simulink library "variant_3_WEC_Sim_Lib"  (R2014a)
settings: Solver=ode45  StartTime=0.0  StopTime=10.0  RelTol=1e-3
undefined symbols (not defined in the file): body, constraint, pto, simu, waves, X, Y, Z
libraries: nesl_utility x56, sm_lib x43
(part 1 of 2)
settings Model: ForwardingTableString=||__slOldName__||WECSim_Lib/Joints/Translational (heave) PCC||__slNewName__||WECSim_Lib/Joints/Translational (Heave) PCC  Creator=cmichel  LastModifiedBy=cmichel

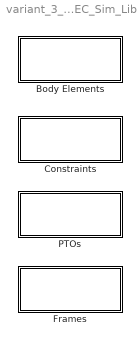
== system variant_3_WEC_Sim_Lib ==
  Body Elements : Subsystem
      mask Display: text(0,0,' ')
  Constraints : Subsystem
      mask Display: text(0,0,' ')
  Frames : Subsystem
      mask Display: text(0,0,' ')
  PTOs : Subsystem
      mask Display: text(0,0,' ')

== system variant_3_WEC_Sim_Lib/Body Elements ==
  Rigid Body : Subsystem  mask(BodyElements){body=body(1)}
      mask prompts: body "Body Name:"
      mask help: This block represents a rigid body. The variable name input below must be 'body(i)' where i=1,2,...
      mask init:
      | if exist('body','var')
      |     h=[gcb '/Structure/Body Properties'];
      |     geomFile=body.geom.file;
      |     set_param(h,'ExtGeomFileName',geomFile);
      |     h=[gcb '/To Workspace'];
      |     responseName=[body.name '_out'];
      |     set_param(h,'VariableName',responseName);
      | end
      | clear bc h geomFile responseName
      settings: AttributesFormatString=%<body>

== system variant_3_WEC_Sim_Lib/Constraints ==
  Fixed : Subsystem  mask(Constraints){constraint=constraint(1)}
      mask prompts: constraint "Constraint Name:"
      mask help:
      | Does not allow any motion. The variable name input below must be 'constraint(i)' where i=1,2,...
      |
      | constraint(i) must be defined in the input file with the following fields:
      |     .name   = a string
      |
      | The name string is used as the variable name for the output power and as such must comply with all of Matlab's variable naming rules.
      mask init:
      | if exist('constraint','var')
      |     h=[gcb '/output'];
      |     responseName=[constraint.name '_out'];
      |     set_param(h,'VariableName',responseName);
      | end
      | 
      | if constraint.loc == [9999 9999 9999]
      |     pto.loc = [0 0 0];
      | end
      settings: AttributesFormatString=%<constraint>
  Floating : Subsystem  mask(Constraints){constraint=constraint(1)}
      mask prompts: constraint "Constraint Name:"
      mask help:
      | Allows body to be free floating (motion in Surge, Heave, and Pitch). The variable name input below must be 'constraint(i)' where i=1,2,...
      |
      | constraint(i) must be defined in the input file with the following fields:
      |     .name   = a string
      |
      | The name string is used as the variable name for the output power and as such must comply with all of Matlab's variable naming rules.
      mask init: same as variant_3_WEC_Sim_Lib/Constraints/Fixed
      settings: AttributesFormatString=%<constraint>
  Heave : Subsystem  mask(Constraints){constraint=constraint(1)}
      mask prompts: constraint "Constraint Name:"
      mask help:
      | Constrains motion to Heave translation only.The variable name input below must be 'constraint(i)' where i=1,2,...
      |
      | constraint(i) must be defined in the input file with the following fields:
      |     .name   = a string
      |
      | The name string is used as the variable name for the output power and as such must comply with all of Matlab's variable naming rules.
      mask init: same as variant_3_WEC_Sim_Lib/Constraints/Fixed
      settings: AttributesFormatString=%<constraint>
  Pitch : Subsystem  mask(Constraints){constraint=constraint(1)}
      mask prompts: constraint "Constraint Name:"
      mask help:
      | Constrains motion to Pitch rotation only. The variable name input below must be 'constraint(i)' where i=1,2,...
      |
      | constraint(i) must be defined in the input file with the following fields:
      |     .name   = a string
      |     .loc    = a 3x1 vector [x y z] in m
      |
      | The name string is used as the variable name for the output power and as such must comply with all of Matlab's variable naming rules.
      mask init:
      | if exist('constraint','var')
      |     h=[gcb '/output'];
      |     responseName=[constraint.name '_out'];
      |     set_param(h,'VariableName',responseName);
      | end
      settings: AttributesFormatString=%<constraint>
  Surge : Subsystem  mask(Constraints){constraint=constraint(1)}
      mask prompts: constraint "Constraint Name:"
      mask help:
      | Constrains motion to Surge translation only.The variable name input below must be 'constraint(i)' where i=1,2,...
      |
      | constraint(i) must be defined in the input file with the following fields:
      |     .name   = a string
      |
      | The name string is used as the variable name for the output power and as such must comply with all of Matlab's variable naming rules.
      mask init: same as variant_3_WEC_Sim_Lib/Constraints/Fixed
      settings: AttributesFormatString=%<constraint>

== system variant_3_WEC_Sim_Lib/Frames ==
  Global Reference Frame : Subsystem  mask(Frames){waves=waves, simu=simu}
      mask prompts: waves "Wave Class Name"; simu "Simulation Class Name"
      mask help:
      | This block contains Global References, including solver configurations, free surface and seabed description, and simulation time.
      | It uses the following fields from the Simulation and Wave classes:
      |
      | Simulation Class:
      |     .endTime
      |     .dt
      |     .domainSize
      |
      | Wave Class:
      |     .waterDepth

== system variant_3_WEC_Sim_Lib/PTOs ==
  External PTO Rotational (Local RY) : Subsystem  mask(External PTO){pto=pto(1)}
      mask prompts: pto "PTO Name:"
      mask help:
      | This PTO constrains the follower (F) to only rotate about the Y-axis of the base (B).
      | The joint is externally actuated (user supplied PTO torque). The joint outputs position and velocity for the user to use in calculating PTO torque.
      mask init:
      | if exist('pto','var')
      |     h=[gcb '/output'];
      |     responseName=[pto.name '_out'];
      |     set_param(h,'VariableName',responseName);
      | end
      settings: AttributesFormatString=%<pto>
  External PTO Translational (Local X) : Subsystem  mask(External PTO){pto=pto(1)}
      mask prompts: pto "PTO Name:"
      mask help:
      | This PTO constrains the follower (F) to only move along the X-direction of the base (B).
      | The joint is externally actuated (user supplied PTO force). The joint outputs position and velocity for the user to use in calculating PTO forces.
      mask init:
      | if exist('pto','var')
      |     h=[gcb '/output'];
      |     responseName=[pto.name '_out'];
      |     set_param(h,'VariableName',responseName);
      | end
      | 
      | if pto.loc == [9999 9999 9999]
      |     pto.loc = [0 0 0];
      | end
      settings: AttributesFormatString=%<pto>
  External PTO Translational (Local Z) : Subsystem  mask(External PTO){pto=pto(1)}
      mask prompts: pto "PTO Name:"
      mask help:
      | This PTO constrains the follower (F) to only move along the Z-direction of the base (B).
      | The joint is externally actuated (user supplied PTO force). The joint outputs position and velocity for the user to use in calculating PTO force.
      mask init:
      | if exist('pto','var')
      |     h=[gcb '/output'];
      |     responseName=[pto.name '_out'];
      |     set_param(h,'VariableName',responseName);
      | end
      | 
      | if pto.loc == [9999 9999 9999]
      |     pto.loc = [0 0 0];
      | end
      settings: AttributesFormatString=%<pto>
  Rotational PTO (Local RY) : Subsystem  mask(PTO){pto=pto(1)}
      mask prompts: pto "PTO Name:"
      mask help:
      | This PTO constrains the follower (F) to only rotate about the Y-axis of the base (B), and applies a PTO stiffness and damping value. The variable name input below must be 'pto(i)' where i=1,2,...
      |
      | pto(i) must be defined in the input file with the following fields:
      |     .name   = a string
      |     .k      = a scalar in N*m/radians
      |     .c      = a scalar in N*m/(radians/s)
      |     .loc    = a 3x1 vector [x y z] in m
      |
      | The name string is used as the variable name for the output power and as such must comply with all of Matlab's variable naming rules.
      mask init:
      | if exist('pto','var')
      |     h=[gcb '/output'];
      |     responseName=[pto.name '_out'];
      |     set_param(h,'VariableName',responseName);
      | end
      settings: AttributesFormatString=%<pto>
  Translational PTO (Local X) : Subsystem  mask(PTO){pto=pto(1)}
      mask prompts: pto "PTO Name:"
      mask help:
      | This PTO constrains the follower (F) to only move along the X-direction of the base (B), and applies a PTO stiffness and damping value. The variable name input below must be 'pto(i)' where i=1,2,...
      |
      | pto(i) must be defined in the input file with the following fields:
      |     .name   = a string
      |     .k      = a scalar in N/m
      |     .c      = a scalar in N/(m/s)
      |
      | The name string is used as the variable name for the output power and as such must comply with all of Matlab's variable naming rules.
      mask init:
      | if exist('pto','var')
      |     h=[gcb '/output'];
      |     responseName=[pto.name '_out'];
      |     set_param(h,'VariableName',responseName);
      | end
      | 
      | if pto.loc == [9999 9999 9999]
      |     pto.loc = [0 0 0];
      | end
      settings: AttributesFormatString=%<pto>
  Translational PTO (Local Z) : Subsystem  mask(PTO){pto=pto(1)}
      mask prompts: pto "PTO Name:"
      mask help:
      | This PTO constrains the follower (F) to only move along the Z-direction of the base (B), and applies a PTO stiffness and damping value. The variable name input below must be 'pto(i)' where i=1,2,...
      |
      | pto(i) must be defined in the input file with the following fields:
      |     .name   = a string
      |     .k      = a scalar in N/m
      |     .c      = a scalar in N/(m/s)
      |
      | The name string is used as the variable name for the output power and as such must comply with all of Matlab's variable naming rules.
      mask init:
      | if exist('pto','var')
      |     h=[gcb '/output'];
      |     responseName=[pto.name '_out'];
      |     set_param(h,'VariableName',responseName);
      | end
      | 
      | if pto.loc == [9999 9999 9999]
      |     pto.loc = [0 0 0];
      | end
      settings: AttributesFormatString=%<pto>

== system variant_3_WEC_Sim_Lib/Body Elements/Rigid Body ==
  Bus Creator : BusCreator  Inputs=5
  Bus Creator1 : BusCreator  Inputs=3
  Bus Selector : BusSelector  OutputSignals=disp,vel,accel
  Bus Selector1 : BusSelector  OutputSignals=F_Excitation,F_Restoring,F_Viscous,F_Mooring,F_Radiation
  Hydrostatic Restoring Force Calculation : Subsystem
  Mooring Force Calculation (Map) : Subsystem
  Structure : Subsystem
  Sum : Sum  Inputs=+----
  To Workspace : ToWorkspace  VariableName=Flap_out  SaveFormat=Structure With Time  SampleTime=-1
  Viscous Damping Force Calculation : Subsystem
  Wave Diffraction and Excitation Force Calculation : Subsystem
  Wave Radiation Forces Calculation : Subsystem
  Conn : PMIOPort  Port=1  Side=Right
  wires:
  Sum/1 -> Bus Creator1/2, Structure/1(F_vector)
  Bus Selector/1 -> Mooring Force Calculation (Map)/1(Displacement), Hydrostatic Restoring Force Calculation/1(Displacement)  "<disp>"
  Bus Selector/2 -> Mooring Force Calculation (Map)/2(Velocity), Viscous Damping Force Calculation/1(Velocity), Wave Radiation Forces Calculation/1(Velocity)  "<vel>"
  Structure/1(Response) -> Bus Selector/1, Bus Creator1/1
  Bus Creator/1 -> Bus Creator1/3, Bus Selector1/1
  Bus Creator1/1 -> To Workspace/1
  Bus Selector/3 -> Wave Radiation Forces Calculation/2(Acceleration)  "<accel>"
  Mooring Force Calculation (Map)/1(F_Mooring) -> Bus Creator/5
  Viscous Damping Force Calculation/1(F_Viscous) -> Bus Creator/4
  Hydrostatic Restoring Force Calculation/1(F_Restoring) -> Bus Creator/3
  Wave Radiation Forces Calculation/1(F_Radiation) -> Bus Creator/2
  Wave Diffraction and Excitation Force Calculation/1(F_Excitation) -> Bus Creator/1
  Bus Selector1/1 -> Sum/1  "<F_Excitation>"
  Bus Selector1/2 -> Sum/2  "<F_Restoring>"
  Bus Selector1/3 -> Sum/3  "<F_Viscous>"
  Bus Selector1/4 -> Sum/4  "<F_Mooring>"
  Bus Selector1/5 -> Sum/5  "<F_Radiation>"
  connections:
  Structure/RConn1 -- Conn/RConn1

== system variant_3_WEC_Sim_Lib/Constraints/Fixed ==
  Mux : Mux  Inputs=2
  PSS : nesl_utility/PS-Simulink Converter  PhysicalDomain=network_engine_domain  SubClassName=ps_output  LeftPortType=input  RightPortType=output  PseudoPeriodic=off  Frequencies=[]  Unit=1  AffineConversion=off
  PSS1 : nesl_utility/PS-Simulink Converter  PhysicalDomain=network_engine_domain  SubClassName=ps_output  LeftPortType=input  RightPortType=output  PseudoPeriodic=off  Frequencies=[]  Unit=1  AffineConversion=off
  Rigid Transform : sm_lib/Frames and Transforms/Rigid Transform  TranslationMethod=Cartesian  TranslationLengthUnit=m  TranslationStandardAxis=+Z  TranslationStandardOffset=0  TranslationCartesianOffset=constraint.loc  TranslationROffset=0  TranslationROffsetUnits=m  TranslationZOffset=0  TranslationZOffsetUnits=m  TranslationThetaOffset=0  TranslationThetaOffsetUnits=deg  RotationMethod=None  RotationAngleUnits=deg  RotationStandardAxis=+X  RotationAngle=90  RotationArbitraryAxis=[0 0 1]  FollAlignAxisA=+X  BaseAlignAxisA=+Y  FollAlignAxisB=+Y  BaseAlignAxisB=+Z  BlockFunction=simmechanics.library.frames_transforms.rigid_transform
  Rigid Transform1 : sm_lib/Frames and Transforms/Rigid Transform  TranslationMethod=Cartesian  TranslationLengthUnit=m  TranslationStandardAxis=+Z  TranslationStandardOffset=0  TranslationCartesianOffset=constraint.loc  TranslationROffset=0  TranslationROffsetUnits=m  TranslationZOffset=0  TranslationZOffsetUnits=m  TranslationThetaOffset=0  TranslationThetaOffsetUnits=deg  RotationMethod=None  RotationAngleUnits=deg  RotationStandardAxis=+X  RotationAngle=90  RotationArbitraryAxis=[0 0 1]  FollAlignAxisA=+X  BaseAlignAxisA=+Y  FollAlignAxisB=+Y  BaseAlignAxisB=+Z  BlockFunction=simmechanics.library.frames_transforms.rigid_transform
  Weld Joint : sm_lib/Joints/Weld Joint  SenseConstraintForce=on  SenseConstraintForceX=off  SenseConstraintForceY=off  SenseConstraintForceZ=off  SenseConstraintTorque=on  SenseConstraintTorqueX=off  SenseConstraintTorqueY=off  SenseConstraintTorqueZ=off  SenseTotalForce=off  SenseTotalForceX=off  SenseTotalForceY=off  SenseTotalForceZ=off  SenseTotalTorque=off  SenseTotalTorqueX=off  SenseTotalTorqueY=off  SenseTotalTorqueZ=off  CompositeWrenchDir=BaseOnFollower  CompositeWrenchFrame=BaseFrame  BlockFunction=simmechanics.library.joints.weld_joint
  output : ToWorkspace  VariableName=Constraint1_out  SaveFormat=Structure With Time  SampleTime=-1
  B : PMIOPort  Port=1  Side=Left
  F : PMIOPort  Port=2  Side=Right
  wires:
  PSS/1 -> Mux/1
  PSS1/1 -> Mux/2
  Mux/1 -> output/1  "Constraint Forces"
  connections:
  PSS1/LConn1 -- Weld Joint/RConn3
  PSS/LConn1 -- Weld Joint/RConn2
  Weld Joint/RConn1 -- Rigid Transform1/RConn1
  Rigid Transform1/LConn1 -- F/RConn1
  Rigid Transform/RConn1 -- Weld Joint/LConn1
  Rigid Transform/LConn1 -- B/RConn1

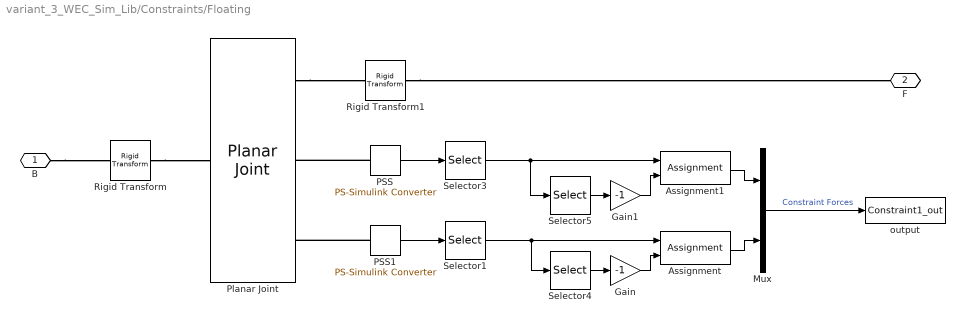
== system variant_3_WEC_Sim_Lib/Constraints/Floating ==
  Assignment : Assignment  DiagnosticForDimensions=Warning  Indices=2
  Assignment1 : Assignment  DiagnosticForDimensions=Warning  Indices=2
  Gain : Gain  Gain=-1
  Gain1 : Gain  Gain=-1
  Mux : Mux  Inputs=2
  PSS : nesl_utility/PS-Simulink Converter  PhysicalDomain=network_engine_domain  SubClassName=ps_output  LeftPortType=input  RightPortType=output  PseudoPeriodic=off  Frequencies=[]  Unit=1  AffineConversion=off
  PSS1 : nesl_utility/PS-Simulink Converter  PhysicalDomain=network_engine_domain  SubClassName=ps_output  LeftPortType=input  RightPortType=output  PseudoPeriodic=off  Frequencies=[]  Unit=1  AffineConversion=off
  Planar Joint : sm_lib/Joints/Planar Joint  SenseConstraintForce=on  SenseConstraintForceX=off  SenseConstraintForceY=off  SenseConstraintForceZ=off  SenseConstraintTorque=on  SenseConstraintTorqueX=off  SenseConstraintTorqueY=off  SenseConstraintTorqueZ=off  SenseTotalForce=off  SenseTotalForceX=off  SenseTotalForceY=off  SenseTotalForceZ=off  SenseTotalTorque=off  SenseTotalTorqueX=off  SenseTotalTorqueY=off  SenseTotalTorqueZ=off  CompositeWrenchDir=BaseOnFollower  CompositeWrenchFrame=BaseFrame  PxEquilibriumPosition=0  PxEquilibriumPositionUnits=m  PxSpringStiffness=0  PxSpringStiffnessUnits=N/m  PxDampingCoefficient=0  PxDampingCoefficientUnits=N/(m/s)  PxTorqueActuationMode=NoTorque  PxMotionActuationMode=ComputedMotion  PxSensePosition=off  PxSenseVelocity=off  PxSenseAcceleration=off  PxSenseTorqueForce=off  PxPositionTargetValue=0  PxPositionTargetValueUnits=m  PxPositionTargetSpecify=off  PxPositionTargetPriority=High  PxVelocityTargetValue=0  PxVelocityTargetValueUnits=m/s  PxVelocityTargetSpecify=off  PxVelocityTargetPriority=High  PyEquilibriumPosition=0  PyEquilibriumPositionUnits=m  PySpringStiffness=0  PySpringStiffnessUnits=N/m  PyDampingCoefficient=0  PyDampingCoefficientUnits=N/(m/s)  PyTorqueActuationMode=NoTorque  PyMotionActuationMode=ComputedMotion  PySensePosition=off  PySenseVelocity=off  PySenseAcceleration=off  PySenseTorqueForce=off  PyPositionTargetValue=0  PyPositionTargetValueUnits=m  PyPositionTargetSpecify=off  PyPositionTargetPriority=High  PyVelocityTargetValue=0  PyVelocityTargetValueUnits=m/s  PyVelocityTargetSpecify=off  PyVelocityTargetPriority=High  RzEquilibriumPosition=0  RzEquilibriumPositionUnits=deg  RzSpringStiffness=0  RzSpringStiffnessUnits=N*m/deg  RzDampingCoefficient=0  RzDampingCoefficientUnits=N*m/(deg/s)  RzTorqueActuationMode=NoTorque  RzMotionActuationMode=ComputedMotion  RzSensePosition=off  RzSenseVelocity=off  RzSenseAcceleration=off  RzSenseTorqueForce=off  RzPositionTargetValue=0  RzPositionTargetValueUnits=deg  RzPositionTargetSpecify=off  RzPositionTargetPriority=High  RzVelocityTargetValue=0  RzVelocityTargetValueUnits=deg/s  RzVelocityTargetSpecify=off  RzVelocityTargetPriority=High  BlockFunction=simmechanics.library.joints.planar_joint
  Rigid Transform : sm_lib/Frames and Transforms/Rigid Transform  TranslationMethod=Cartesian  TranslationLengthUnit=m  TranslationStandardAxis=+Z  TranslationStandardOffset=0  TranslationCartesianOffset=constraint.loc  TranslationROffset=0  TranslationROffsetUnits=m  TranslationZOffset=0  TranslationZOffsetUnits=m  TranslationThetaOffset=0  TranslationThetaOffsetUnits=deg  RotationMethod=StandardAxis  RotationAngleUnits=deg  RotationStandardAxis=+X  RotationAngle=90  RotationArbitraryAxis=[0 0 1]  FollAlignAxisA=+X  BaseAlignAxisA=+Y  FollAlignAxisB=+Y  BaseAlignAxisB=+Z  BlockFunction=simmechanics.library.frames_transforms.rigid_transform
  Rigid Transform1 : sm_lib/Frames and Transforms/Rigid Transform  TranslationMethod=Cartesian  TranslationLengthUnit=m  TranslationStandardAxis=+Z  TranslationStandardOffset=0  TranslationCartesianOffset=constraint.loc  TranslationROffset=0  TranslationROffsetUnits=m  TranslationZOffset=0  TranslationZOffsetUnits=m  TranslationThetaOffset=0  TranslationThetaOffsetUnits=deg  RotationMethod=StandardAxis  RotationAngleUnits=deg  RotationStandardAxis=+X  RotationAngle=90  RotationArbitraryAxis=[0 0 1]  FollAlignAxisA=+X  BaseAlignAxisA=+Y  FollAlignAxisB=+Y  BaseAlignAxisB=+Z  BlockFunction=simmechanics.library.frames_transforms.rigid_transform
  Selector1 : Selector  InputPortWidth=3  Indices=[1 3 2]
  Selector3 : Selector  InputPortWidth=3  Indices=[1 3 2]
  Selector4 : Selector  InputPortWidth=3  Indices=[2]
  Selector5 : Selector  InputPortWidth=3  Indices=[2]
  output : ToWorkspace  VariableName=Constraint1_out  SaveFormat=Structure With Time  SampleTime=-1
  B : PMIOPort  Port=1  Side=Left
  F : PMIOPort  Port=2  Side=Right
  wires:
  Mux/1 -> output/1  "Constraint Forces"
  Selector1/1 -> Assignment/1, Selector4/1
  Selector4/1 -> Gain/1
  Gain/1 -> Assignment/2
  Selector3/1 -> Assignment1/1, Selector5/1
  Selector5/1 -> Gain1/1
  Gain1/1 -> Assignment1/2
  PSS1/1 -> Selector1/1
  PSS/1 -> Selector3/1
  Assignment1/1 -> Mux/1
  Assignment/1 -> Mux/2
  connections:
  Rigid Transform1/LConn1 -- F/RConn1
  Planar Joint/RConn1 -- Rigid Transform1/RConn1
  Rigid Transform/RConn1 -- Planar Joint/LConn1
  B/RConn1 -- Rigid Transform/LConn1
  PSS/LConn1 -- Planar Joint/RConn2
  PSS1/LConn1 -- Planar Joint/RConn3

== system variant_3_WEC_Sim_Lib/Constraints/Heave ==
  Mux : Mux  Inputs=2
  PSS : nesl_utility/PS-Simulink Converter  PhysicalDomain=network_engine_domain  SubClassName=ps_output  LeftPortType=input  RightPortType=output  PseudoPeriodic=off  Frequencies=[]  Unit=1  AffineConversion=off
  PSS1 : nesl_utility/PS-Simulink Converter  PhysicalDomain=network_engine_domain  SubClassName=ps_output  LeftPortType=input  RightPortType=output  PseudoPeriodic=off  Frequencies=[]  Unit=1  AffineConversion=off
  Rigid Transform : sm_lib/Frames and Transforms/Rigid Transform  TranslationMethod=Cartesian  TranslationLengthUnit=m  TranslationStandardAxis=+Z  TranslationStandardOffset=0  TranslationCartesianOffset=constraint.loc  TranslationROffset=0  TranslationROffsetUnits=m  TranslationZOffset=0  TranslationZOffsetUnits=m  TranslationThetaOffset=0  TranslationThetaOffsetUnits=deg  RotationMethod=None  RotationAngleUnits=deg  RotationStandardAxis=+X  RotationAngle=90  RotationArbitraryAxis=[0 0 1]  FollAlignAxisA=+X  BaseAlignAxisA=+Y  FollAlignAxisB=+Y  BaseAlignAxisB=+Z  BlockFunction=simmechanics.library.frames_transforms.rigid_transform
  Rigid Transform1 : sm_lib/Frames and Transforms/Rigid Transform  TranslationMethod=Cartesian  TranslationLengthUnit=m  TranslationStandardAxis=+Z  TranslationStandardOffset=0  TranslationCartesianOffset=constraint.loc  TranslationROffset=0  TranslationROffsetUnits=m  TranslationZOffset=0  TranslationZOffsetUnits=m  TranslationThetaOffset=0  TranslationThetaOffsetUnits=deg  RotationMethod=None  RotationAngleUnits=deg  RotationStandardAxis=+X  RotationAngle=90  RotationArbitraryAxis=[0 0 1]  FollAlignAxisA=+X  BaseAlignAxisA=+Y  FollAlignAxisB=+Y  BaseAlignAxisB=+Z  BlockFunction=simmechanics.library.frames_transforms.rigid_transform
  Translational Constraint (Prismatic Joint) : sm_lib/Joints/Prismatic Joint  SenseConstraintForce=on  SenseConstraintForceX=off  SenseConstraintForceY=off  SenseConstraintForceZ=off  SenseConstraintTorque=on  SenseConstraintTorqueX=off  SenseConstraintTorqueY=off  SenseConstraintTorqueZ=off  SenseTotalForce=off  SenseTotalForceX=off  SenseTotalForceY=off  SenseTotalForceZ=off  SenseTotalTorque=off  SenseTotalTorqueX=off  SenseTotalTorqueY=off  SenseTotalTorqueZ=off  CompositeWrenchDir=BaseOnFollower  CompositeWrenchFrame=BaseFrame  EquilibriumPosition=0  EquilibriumPositionUnits=m  SpringStiffness=0  SpringStiffnessUnits=N/m  DampingCoefficient=0  DampingCoefficientUnits=N/(m/s)  TorqueActuationMode=NoTorque  MotionActuationMode=ComputedMotion  SensePosition=off  SenseVelocity=off  SenseAcceleration=off  SenseTorqueForce=off  PositionTargetValue=0  PositionTargetValueUnits=m  PositionTargetSpecify=off  PositionTargetPriority=High  VelocityTargetValue=0  VelocityTargetValueUnits=m/s  VelocityTargetSpecify=off  VelocityTargetPriority=High  BlockFunction=simmechanics.library.joints.prismatic_joint
  output : ToWorkspace  VariableName=Constraint1_out  SaveFormat=Structure With Time  SampleTime=-1
  F : PMIOPort  Port=1  Side=Right
  B : PMIOPort  Port=2  Side=Left
  wires:
  PSS/1 -> Mux/1
  PSS1/1 -> Mux/2
  Mux/1 -> output/1  "Constraint Forces"
  connections:
  PSS/LConn1 -- Translational Constraint (Prismatic Joint)/RConn2
  PSS1/LConn1 -- Translational Constraint (Prismatic Joint)/RConn3
  Translational Constraint (Prismatic Joint)/RConn1 -- Rigid Transform1/RConn1
  Rigid Transform1/LConn1 -- F/RConn1
  B/RConn1 -- Rigid Transform/LConn1
  Rigid Transform/RConn1 -- Translational Constraint (Prismatic Joint)/LConn1

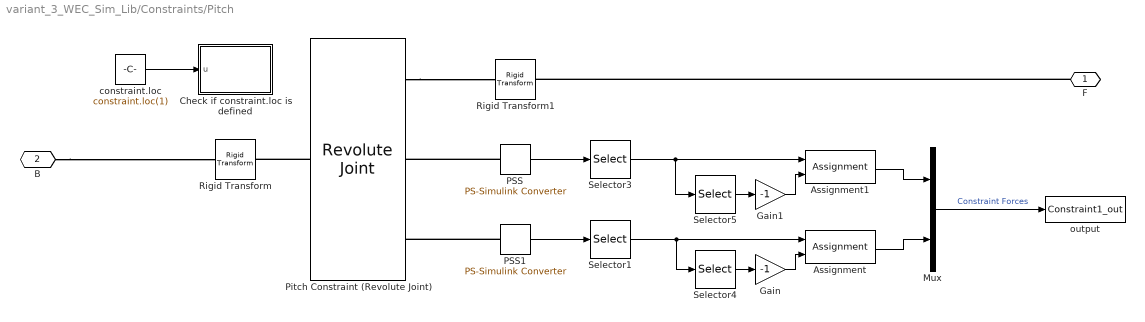
== system variant_3_WEC_Sim_Lib/Constraints/Pitch ==
  Assignment : Assignment  DiagnosticForDimensions=Warning  Indices=2
  Assignment1 : Assignment  DiagnosticForDimensions=Warning  Indices=2
  "Check if constraint.loc is defined " : MATLAB Function  TreatAsAtomicUnit=on
  Gain : Gain  Gain=-1
  Gain1 : Gain  Gain=-1
  Mux : Mux  Inputs=2
  PSS : nesl_utility/PS-Simulink Converter  PhysicalDomain=network_engine_domain  SubClassName=ps_output  LeftPortType=input  RightPortType=output  PseudoPeriodic=off  Frequencies=[]  Unit=1  AffineConversion=off
  PSS1 : nesl_utility/PS-Simulink Converter  PhysicalDomain=network_engine_domain  SubClassName=ps_output  LeftPortType=input  RightPortType=output  PseudoPeriodic=off  Frequencies=[]  Unit=1  AffineConversion=off
  Pitch Constraint (Revolute Joint) : sm_lib/Joints/Revolute Joint  SenseConstraintForce=on  SenseConstraintForceX=off  SenseConstraintForceY=off  SenseConstraintForceZ=off  SenseConstraintTorque=on  SenseConstraintTorqueX=off  SenseConstraintTorqueY=off  SenseConstraintTorqueZ=off  SenseTotalForce=off  SenseTotalForceX=off  SenseTotalForceY=off  SenseTotalForceZ=off  SenseTotalTorque=off  SenseTotalTorqueX=off  SenseTotalTorqueY=off  SenseTotalTorqueZ=off  CompositeWrenchDir=BaseOnFollower  CompositeWrenchFrame=BaseFrame  EquilibriumPosition=0  EquilibriumPositionUnits=deg  SpringStiffness=0  SpringStiffnessUnits=N*m/deg  DampingCoefficient=0  DampingCoefficientUnits=N*m/(rad/s)  TorqueActuationMode=NoTorque  MotionActuationMode=ComputedMotion  SensePosition=off  SenseVelocity=off  SenseAcceleration=off  SenseTorqueForce=off  PositionTargetValue=0  PositionTargetValueUnits=deg  PositionTargetSpecify=off  PositionTargetPriority=High  VelocityTargetValue=0  VelocityTargetValueUnits=deg/s  VelocityTargetSpecify=off  VelocityTargetPriority=High  BlockFunction=simmechanics.library.joints.revolute_joint
  Rigid Transform : sm_lib/Frames and Transforms/Rigid Transform  TranslationMethod=Cartesian  TranslationLengthUnit=m  TranslationStandardAxis=+Z  TranslationStandardOffset=0  TranslationCartesianOffset=constraint.loc  TranslationROffset=0  TranslationROffsetUnits=m  TranslationZOffset=0  TranslationZOffsetUnits=m  TranslationThetaOffset=0  TranslationThetaOffsetUnits=deg  RotationMethod=StandardAxis  RotationAngleUnits=deg  RotationStandardAxis=+X  RotationAngle=90  RotationArbitraryAxis=[0 0 1]  FollAlignAxisA=+X  BaseAlignAxisA=+Y  FollAlignAxisB=+Y  BaseAlignAxisB=+Z  BlockFunction=simmechanics.library.frames_transforms.rigid_transform
  Rigid Transform1 : sm_lib/Frames and Transforms/Rigid Transform  TranslationMethod=Cartesian  TranslationLengthUnit=m  TranslationStandardAxis=+Z  TranslationStandardOffset=0  TranslationCartesianOffset=constraint.loc  TranslationROffset=0  TranslationROffsetUnits=m  TranslationZOffset=0  TranslationZOffsetUnits=m  TranslationThetaOffset=0  TranslationThetaOffsetUnits=deg  RotationMethod=StandardAxis  RotationAngleUnits=deg  RotationStandardAxis=+X  RotationAngle=90  RotationArbitraryAxis=[0 0 1]  FollAlignAxisA=+X  BaseAlignAxisA=+Y  FollAlignAxisB=+Y  BaseAlignAxisB=+Z  BlockFunction=simmechanics.library.frames_transforms.rigid_transform
  Selector1 : Selector  InputPortWidth=3  Indices=[1 3 2]
  Selector3 : Selector  InputPortWidth=3  Indices=[1 3 2]
  Selector4 : Selector  InputPortWidth=3  Indices=[2]
  Selector5 : Selector  InputPortWidth=3  Indices=[2]
  constraint.loc : Constant  Value=constraint.loc(1)  VectorParams1D=off
  output : ToWorkspace  VariableName=Constraint1_out  SaveFormat=Structure With Time  SampleTime=-1
  F : PMIOPort  Port=1  Side=Right
  B : PMIOPort  Port=2  Side=Left
  wires:
  Mux/1 -> output/1  "Constraint Forces"
  constraint.loc/1 -> "Check if constraint.loc is defined "/1(u)
  PSS/1 -> Selector3/1
  PSS1/1 -> Selector1/1
  Selector1/1 -> Assignment/1, Selector4/1
  Selector4/1 -> Gain/1
  Gain/1 -> Assignment/2
  Assignment/1 -> Mux/2
  Selector3/1 -> Assignment1/1, Selector5/1
  Selector5/1 -> Gain1/1
  Gain1/1 -> Assignment1/2
  Assignment1/1 -> Mux/1
  connections:
  Pitch Constraint (Revolute Joint)/LConn1 -- Rigid Transform/RConn1
  Pitch Constraint (Revolute Joint)/RConn1 -- Rigid Transform1/RConn1
  B/RConn1 -- Rigid Transform/LConn1
  F/RConn1 -- Rigid Transform1/LConn1
  PSS/LConn1 -- Pitch Constraint (Revolute Joint)/RConn2
  PSS1/LConn1 -- Pitch Constraint (Revolute Joint)/RConn3

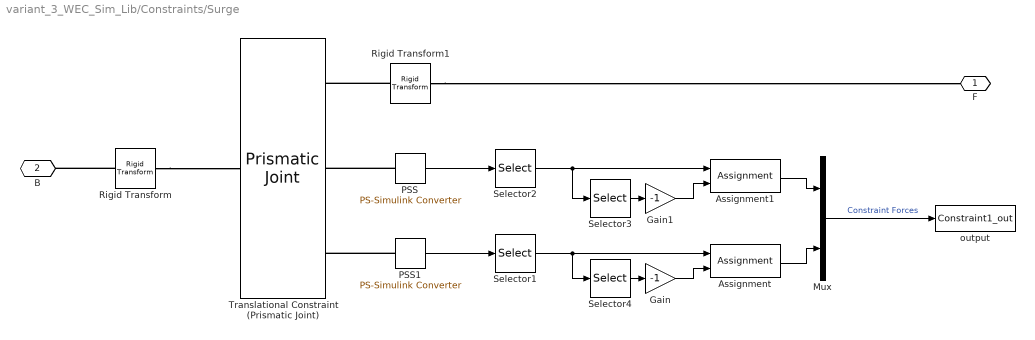
== system variant_3_WEC_Sim_Lib/Constraints/Surge ==
  Assignment : Assignment  DiagnosticForDimensions=Warning  Indices=3
  Assignment1 : Assignment  DiagnosticForDimensions=Warning  Indices=3
  Gain : Gain  Gain=-1
  Gain1 : Gain  Gain=-1
  Mux : Mux  Inputs=2
  PSS : nesl_utility/PS-Simulink Converter  PhysicalDomain=network_engine_domain  SubClassName=ps_output  LeftPortType=input  RightPortType=output  PseudoPeriodic=off  Frequencies=[]  Unit=1  AffineConversion=off
  PSS1 : nesl_utility/PS-Simulink Converter  PhysicalDomain=network_engine_domain  SubClassName=ps_output  LeftPortType=input  RightPortType=output  PseudoPeriodic=off  Frequencies=[]  Unit=1  AffineConversion=off
  Rigid Transform : sm_lib/Frames and Transforms/Rigid Transform  TranslationMethod=Cartesian  TranslationLengthUnit=m  TranslationStandardAxis=+Z  TranslationStandardOffset=0  TranslationCartesianOffset=constraint.loc  TranslationROffset=0  TranslationROffsetUnits=m  TranslationZOffset=0  TranslationZOffsetUnits=m  TranslationThetaOffset=0  TranslationThetaOffsetUnits=deg  RotationMethod=StandardAxis  RotationAngleUnits=deg  RotationStandardAxis=+Y  RotationAngle=90  RotationArbitraryAxis=[0 0 1]  FollAlignAxisA=+X  BaseAlignAxisA=+Y  FollAlignAxisB=+Y  BaseAlignAxisB=+Z  BlockFunction=simmechanics.library.frames_transforms.rigid_transform
  Rigid Transform1 : sm_lib/Frames and Transforms/Rigid Transform  TranslationMethod=Cartesian  TranslationLengthUnit=m  TranslationStandardAxis=+Z  TranslationStandardOffset=0  TranslationCartesianOffset=constraint.loc  TranslationROffset=0  TranslationROffsetUnits=m  TranslationZOffset=0  TranslationZOffsetUnits=m  TranslationThetaOffset=0  TranslationThetaOffsetUnits=deg  RotationMethod=StandardAxis  RotationAngleUnits=deg  RotationStandardAxis=+Y  RotationAngle=90  RotationArbitraryAxis=[0 0 1]  FollAlignAxisA=+X  BaseAlignAxisA=+Y  FollAlignAxisB=+Y  BaseAlignAxisB=+Z  BlockFunction=simmechanics.library.frames_transforms.rigid_transform
  Selector1 : Selector  InputPortWidth=3  Indices=[3 2 1]
  Selector2 : Selector  InputPortWidth=3  Indices=[3 2 1]
  Selector3 : Selector  InputPortWidth=3  Indices=[3]
  Selector4 : Selector  InputPortWidth=3  Indices=[3]
  Translational Constraint (Prismatic Joint) : sm_lib/Joints/Prismatic Joint  SenseConstraintForce=on  SenseConstraintForceX=off  SenseConstraintForceY=off  SenseConstraintForceZ=off  SenseConstraintTorque=on  SenseConstraintTorqueX=off  SenseConstraintTorqueY=off  SenseConstraintTorqueZ=off  SenseTotalForce=off  SenseTotalForceX=off  SenseTotalForceY=off  SenseTotalForceZ=off  SenseTotalTorque=off  SenseTotalTorqueX=off  SenseTotalTorqueY=off  SenseTotalTorqueZ=off  CompositeWrenchDir=BaseOnFollower  CompositeWrenchFrame=BaseFrame  EquilibriumPosition=0  EquilibriumPositionUnits=m  SpringStiffness=0  SpringStiffnessUnits=N/m  DampingCoefficient=0  DampingCoefficientUnits=N/(m/s)  TorqueActuationMode=NoTorque  MotionActuationMode=ComputedMotion  SensePosition=off  SenseVelocity=off  SenseAcceleration=off  SenseTorqueForce=off  PositionTargetValue=0  PositionTargetValueUnits=m  PositionTargetSpecify=off  PositionTargetPriority=High  VelocityTargetValue=0  VelocityTargetValueUnits=m/s  VelocityTargetSpecify=off  VelocityTargetPriority=High  BlockFunction=simmechanics.library.joints.prismatic_joint
  output : ToWorkspace  VariableName=Constraint1_out  SaveFormat=Structure With Time  SampleTime=-1
  F : PMIOPort  Port=1  Side=Right
  B : PMIOPort  Port=2  Side=Left
  wires:
  Mux/1 -> output/1  "Constraint Forces"
  Selector1/1 -> Assignment/1, Selector4/1
  Selector4/1 -> Gain/1
  Gain/1 -> Assignment/2
  PSS1/1 -> Selector1/1
  Selector2/1 -> Assignment1/1, Selector3/1
  Selector3/1 -> Gain1/1
  Gain1/1 -> Assignment1/2
  PSS/1 -> Selector2/1
  Assignment1/1 -> Mux/1
  Assignment/1 -> Mux/2
  connections:
  Rigid Transform1/LConn1 -- F/RConn1
  Rigid Transform1/RConn1 -- Translational Constraint (Prismatic Joint)/RConn1
  Rigid Transform/RConn1 -- Translational Constraint (Prismatic Joint)/LConn1
  Rigid Transform/LConn1 -- B/RConn1
  PSS/LConn1 -- Translational Constraint (Prismatic Joint)/RConn2
  PSS1/LConn1 -- Translational Constraint (Prismatic Joint)/RConn3

== system variant_3_WEC_Sim_Lib/Frames/Global Reference Frame ==
  note: NOTE:Must be a fixed time step solver
      | changed to ode4 (fixed step)
  Clock : Clock
  Mean Free Surface : sm_lib/Body Elements/Solid  InertiaType=Custom  Mass=10^20  MassUnits=kg  CenterOfMass=[0 0 0]  CenterOfMassUnits=m  MomentsOfInertia=[10^20 10^20 10^20]  MomentsOfInertiaUnits=kg*m^2  ProductsOfInertia=[0 0 0]  ProductsOfInertiaUnits=kg*m^2  DensityBased=on  Density=1000  DensityUnits=kg/(m^3)  GraphicType=FromGeometry  MarkerShape=Sphere  MarkerSize=10  MarkerSizeUnits=m  GraphicVisPropType=SimpleVisualProperties  GraphicDiffuseColor=[0.0 0.6 0.8]  GraphicSpecularColor=[0.5 0.5 0.5 1.0]  GraphicAmbientColor=[0.15 0.15 0.15 1.0]  GraphicEmissiveColor=[0.0 0.0 0.0 1.0]  GraphicShininess=75  GraphicOpacity=0.3  GeometryShape=GeneralExtrusion  RectangleSize=[1 1]  RectangleSizeUnits=m  BrickDimensions=[1 1 1]  BrickDimensionUnits=m  CylinderRadius=1  CylinderRadiusUnits=m  CylinderLength=1  CylinderLengthUnits=m  SphereRadius=1  SphereRadiusUnits=m  EllipsoidRadii=[1 1 1]  EllipsoidRadiiUnits=m  ExtrusionCrossSection=[simu.domainSize simu.domainSize; -simu.domainSize simu.domainSize; -simu.domainSize -simu.domainSize; simu.domainSize -simu.domainSize]  ExtrusionCrossSectionUnits=m  ExtrusionLength=simu.domainSize/200  ExtrusionLengthUnits=m  PolygonNumSides=3  PolygonOuterRadius=1  PolygonOuterRadiusUnits=m  ExtGeomFileType=STL  ExtGeomFileUnits=m  RevolutionCrossSection=[1 1; 1 -1; 2 -1; 2 1]  RevolutionCrossSectionUnits=m  RevolutionExtent=Full  RevolutionAngle=180  RevolutionAngleUnits=deg  BlockFunction=simmechanics.library.body_elements.solid
  Mechanism Configuration1 : sm_lib/Utilities/Mechanism Configuration  UniformGravity=Constant  GravityVector=[0 0 0]  GravityUnits=m/s^2  LinearizationDelta=0.001  BlockFunction=simmechanics.library.utilities.mechanism_configuration
  Rigid Transform : sm_lib/Frames and Transforms/Rigid Transform  TranslationMethod=Cartesian  TranslationLengthUnit=m  TranslationStandardAxis=+Z  TranslationStandardOffset=0  TranslationCartesianOffset=[0 0 -waves.waterDepth]  TranslationROffset=0  TranslationROffsetUnits=m  TranslationZOffset=0  TranslationZOffsetUnits=m  TranslationThetaOffset=0  TranslationThetaOffsetUnits=deg  RotationMethod=None  RotationAngleUnits=deg  RotationStandardAxis=+Z  RotationAngle=0  RotationArbitraryAxis=[0 0 1]  FollAlignAxisA=+X  BaseAlignAxisA=+Y  FollAlignAxisB=+Y  BaseAlignAxisB=+Z  BlockFunction=simmechanics.library.frames_transforms.rigid_transform
  Seabed : sm_lib/Body Elements/Solid  InertiaType=Custom  Mass=10^20  MassUnits=kg  CenterOfMass=[0 0 0]  CenterOfMassUnits=m  MomentsOfInertia=[10^20 10^20 10^20]  MomentsOfInertiaUnits=kg*m^2  ProductsOfInertia=[0 0 0]  ProductsOfInertiaUnits=kg*m^2  DensityBased=on  Density=1000  DensityUnits=kg/(m^3)  GraphicType=FromGeometry  MarkerShape=Sphere  MarkerSize=10  MarkerSizeUnits=m  GraphicVisPropType=SimpleVisualProperties  GraphicDiffuseColor=[0.4 0.4 0.0]  GraphicSpecularColor=[0.5 0.5 0.5 1.0]  GraphicAmbientColor=[0.15 0.15 0.15 1.0]  GraphicEmissiveColor=[0.0 0.0 0.0 1.0]  GraphicShininess=75  GraphicOpacity=1  GeometryShape=GeneralExtrusion  RectangleSize=[1 1]  RectangleSizeUnits=m  BrickDimensions=[1 1 1]  BrickDimensionUnits=m  CylinderRadius=1  CylinderRadiusUnits=m  CylinderLength=1  CylinderLengthUnits=m  SphereRadius=1  SphereRadiusUnits=m  EllipsoidRadii=[1 1 1]  EllipsoidRadiiUnits=m  ExtrusionCrossSection=[simu.domainSize simu.domainSize; -simu.domainSize simu.domainSize; -simu.domainSize -simu.domainSize; simu.domainSize -simu.domainSize]  ExtrusionCrossSectionUnits=m  ExtrusionLength=simu.domainSize/100  ExtrusionLengthUnits=m  PolygonNumSides=3  PolygonOuterRadius=1  PolygonOuterRadiusUnits=m  ExtGeomFileType=STL  ExtGeomFileUnits=m  RevolutionCrossSection=[1 1; 1 -1; 2 -1; 2 1]  RevolutionCrossSectionUnits=m  RevolutionExtent=Full  RevolutionAngle=180  RevolutionAngleUnits=deg  BlockFunction=simmechanics.library.body_elements.solid
  Solver Configuration : nesl_utility/Solver Configuration  PhysicalDomain=network_engine_domain  SubClassName=solver  LeftPortType=input  RightPortType=generic  Accelerate=off  Tones=[]  Harmonics=[]  SimulateNoise=off  Profile=off  UseLocalSampling=off  EnableSwitchedLinearOptims=on  FrequencyDomain=off  UseCCode=off  RelTol=0.001  AbsTol=1e-06  MinStep=1e-09  ToWorkspace=off  DoDC=on  ResidualTolerance=1e-9  UseLocalSolver=off  LocalSolverChoice=NE_BACKWARD_EULER_ADVANCER  LocalSolverSampleTime=.001  DoFixedCost=off  MaxNonlinIter=3  MaxModeIter=2  LinearAlgebra=Sparse  DelaysMemoryBudget=1024  AutomaticFiltering=on  FilteringTimeConstant=0.001
  World Frame2 : sm_lib/Frames and Transforms/World Frame  BlockFunction=simmechanics.library.frames_transforms.world_frame
  Conn : PMIOPort  Port=1  Side=Right
  tag scope: Clock=global
  wires:
  Clock/1 -> [Clock]
  connections:
  Mechanism Configuration1/RConn1 -- World Frame2/RConn1 -- Solver Configuration/RConn1 -- Mean Free Surface/RConn1 -- Rigid Transform/LConn1 -- Conn/RConn1
  Seabed/RConn1 -- Rigid Transform/RConn1

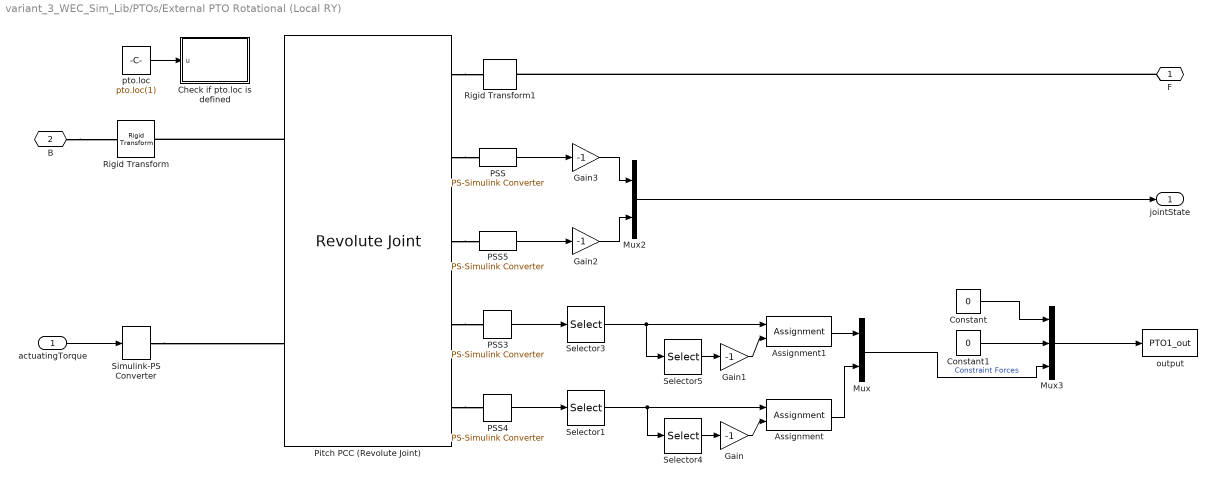
== system variant_3_WEC_Sim_Lib/PTOs/External PTO Rotational (Local RY) ==
  actuatingTorque : Inport
  Assignment : Assignment  DiagnosticForDimensions=Warning  Indices=2
  Assignment1 : Assignment  DiagnosticForDimensions=Warning  Indices=2
  "Check if pto.loc is defined " : MATLAB Function  TreatAsAtomicUnit=on
  Constant : Constant  Value=0
  Constant1 : Constant  Value=0
  Gain{,1..3} (4 alike) : Gain  Gain=-1
  Mux : Mux  Inputs=2
  Mux2 : Mux  Inputs=2
  Mux3 : Mux  Inputs=3
  PSS{,3..5} (4 alike) : nesl_utility/PS-Simulink Converter  PhysicalDomain=network_engine_domain  SubClassName=ps_output  LeftPortType=input  RightPortType=output  PseudoPeriodic=off  Frequencies=[]  Unit=1  AffineConversion=off
  Pitch PCC (Revolute Joint) : sm_lib/Joints/Revolute Joint  SenseConstraintForce=on  SenseConstraintForceX=off  SenseConstraintForceY=off  SenseConstraintForceZ=off  SenseConstraintTorque=on  SenseConstraintTorqueX=off  SenseConstraintTorqueY=off  SenseConstraintTorqueZ=off  SenseTotalForce=off  SenseTotalForceX=off  SenseTotalForceY=off  SenseTotalForceZ=off  SenseTotalTorque=off  SenseTotalTorqueX=off  SenseTotalTorqueY=off  SenseTotalTorqueZ=off  CompositeWrenchDir=BaseOnFollower  CompositeWrenchFrame=BaseFrame  EquilibriumPosition=0  EquilibriumPositionUnits=deg  SpringStiffness=0  SpringStiffnessUnits=N*m/rad  DampingCoefficient=0  DampingCoefficientUnits=N*m/(rad/s)  TorqueActuationMode=InputTorque  MotionActuationMode=ComputedMotion  SensePosition=on  SenseVelocity=on  SenseAcceleration=off  SenseTorqueForce=off  PositionTargetValue=0  PositionTargetValueUnits=deg  PositionTargetSpecify=off  PositionTargetPriority=High  VelocityTargetValue=0  VelocityTargetValueUnits=deg/s  VelocityTargetSpecify=off  VelocityTargetPriority=High  BlockFunction=simmechanics.library.joints.revolute_joint
  Rigid Transform : sm_lib/Frames and Transforms/Rigid Transform  TranslationMethod=Cartesian  TranslationLengthUnit=m  TranslationStandardAxis=+Z  TranslationStandardOffset=0  TranslationCartesianOffset=pto.loc  TranslationROffset=0  TranslationROffsetUnits=m  TranslationZOffset=0  TranslationZOffsetUnits=m  TranslationThetaOffset=0  TranslationThetaOffsetUnits=deg  RotationMethod=StandardAxis  RotationAngleUnits=deg  RotationStandardAxis=+X  RotationAngle=90  RotationArbitraryAxis=[0 0 1]  FollAlignAxisA=+X  BaseAlignAxisA=+Y  FollAlignAxisB=+Y  BaseAlignAxisB=+Z  BlockFunction=simmechanics.library.frames_transforms.rigid_transform
  Rigid Transform1 : sm_lib/Frames and Transforms/Rigid Transform  TranslationMethod=Cartesian  TranslationLengthUnit=m  TranslationStandardAxis=+Z  TranslationStandardOffset=0  TranslationCartesianOffset=pto.loc  TranslationROffset=0  TranslationROffsetUnits=m  TranslationZOffset=0  TranslationZOffsetUnits=m  TranslationThetaOffset=0  TranslationThetaOffsetUnits=deg  RotationMethod=StandardAxis  RotationAngleUnits=deg  RotationStandardAxis=+X  RotationAngle=90  RotationArbitraryAxis=[0 0 1]  FollAlignAxisA=+X  BaseAlignAxisA=+Y  FollAlignAxisB=+Y  BaseAlignAxisB=+Z  BlockFunction=simmechanics.library.frames_transforms.rigid_transform
  Selector1 : Selector  InputPortWidth=3  Indices=[1 3 2]
  Selector3 : Selector  InputPortWidth=3  Indices=[1 3 2]
  Selector4 : Selector  InputPortWidth=3  Indices=[2]
  Selector5 : Selector  InputPortWidth=3  Indices=[2]
  Simulink-PS Converter : nesl_utility/Simulink-PS Converter  PhysicalDomain=network_engine_domain  SubClassName=ps_input  LeftPortType=input  RightPortType=output  PseudoPeriodic=off  Frequencies=[]  NoiseDistribution=none  NoiseParameters=[]  Unit=1  AffineConversion=off  InputFiltering=off  SimscapeFilterOrder=1  InputFilterTimeConstant=0.001  UdotUserProvided=1
  output : ToWorkspace  VariableName=PTO1_out  SaveFormat=Structure With Time  SampleTime=-1
  pto.loc : Constant  Value=pto.loc(1)  VectorParams1D=off
  F : PMIOPort  Port=1  Side=Right
  B : PMIOPort  Port=2  Side=Left
  jointState : Outport
  wires:
  pto.loc/1 -> "Check if pto.loc is defined "/1(u)
  PSS5/1 -> Gain2/1
  PSS/1 -> Gain3/1
  Mux2/1 -> jointState/1
  actuatingTorque/1 -> Simulink-PS Converter/1
  PSS3/1 -> Selector3/1
  PSS4/1 -> Selector1/1
  Mux/1 -> Mux3/3  "Constraint Forces"
  Selector1/1 -> Assignment/1, Selector4/1
  Selector4/1 -> Gain/1
  Gain/1 -> Assignment/2
  Assignment/1 -> Mux/2
  Selector3/1 -> Assignment1/1, Selector5/1
  Selector5/1 -> Gain1/1
  Gain1/1 -> Assignment1/2
  Assignment1/1 -> Mux/1
  Gain3/1 -> Mux2/1
  Gain2/1 -> Mux2/2
  Constant/1 -> Mux3/1
  Constant1/1 -> Mux3/2
  Mux3/1 -> output/1
  connections:
  F/RConn1 -- Rigid Transform1/LConn1
  B/RConn1 -- Rigid Transform/LConn1
  Pitch PCC (Revolute Joint)/RConn1 -- Rigid Transform1/RConn1
  Pitch PCC (Revolute Joint)/LConn1 -- Rigid Transform/RConn1
  Pitch PCC (Revolute Joint)/RConn2 -- PSS/LConn1
  Pitch PCC (Revolute Joint)/RConn3 -- PSS5/LConn1
  Simulink-PS Converter/RConn1 -- Pitch PCC (Revolute Joint)/LConn2
  Pitch PCC (Revolute Joint)/RConn4 -- PSS3/LConn1
  Pitch PCC (Revolute Joint)/RConn5 -- PSS4/LConn1

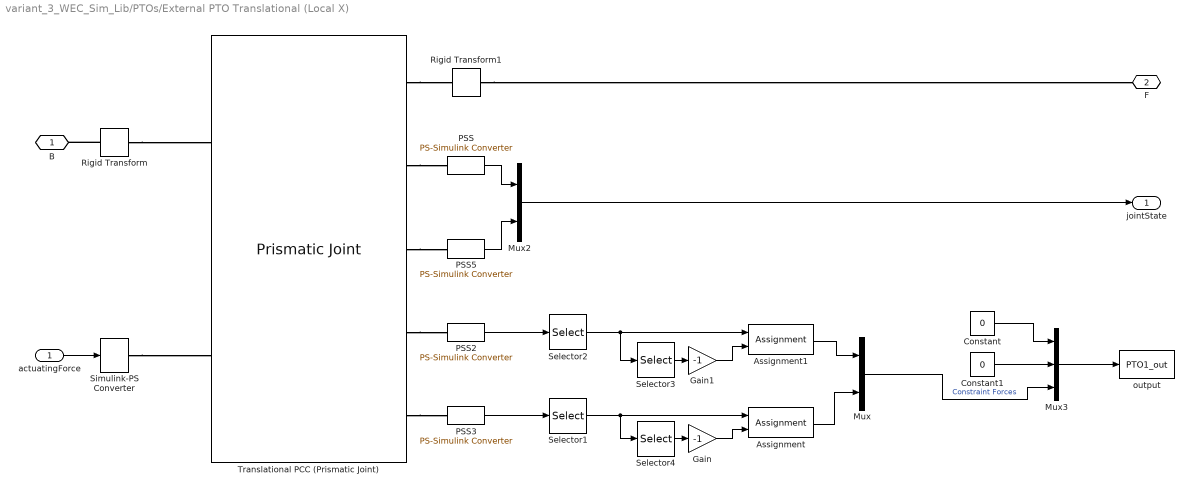
== system variant_3_WEC_Sim_Lib/PTOs/External PTO Translational (Local X) ==
  actuatingForce : Inport
  Assignment : Assignment  DiagnosticForDimensions=Warning  Indices=3
  Assignment1 : Assignment  DiagnosticForDimensions=Warning  Indices=3
  Constant : Constant  Value=0
  Constant1 : Constant  Value=0
  Gain : Gain  Gain=-1
  Gain1 : Gain  Gain=-1
  Mux : Mux  Inputs=2
  Mux2 : Mux  Inputs=2
  Mux3 : Mux  Inputs=3
  PSS{,2..3,5} (4 alike) : nesl_utility/PS-Simulink Converter  PhysicalDomain=network_engine_domain  SubClassName=ps_output  LeftPortType=input  RightPortType=output  PseudoPeriodic=off  Frequencies=[]  Unit=1  AffineConversion=off
  Rigid Transform : sm_lib/Frames and Transforms/Rigid Transform  TranslationMethod=None  TranslationLengthUnit=m  TranslationStandardAxis=+Z  TranslationStandardOffset=0  TranslationCartesianOffset=[0 0 0]  TranslationROffset=0  TranslationROffsetUnits=m  TranslationZOffset=0  TranslationZOffsetUnits=m  TranslationThetaOffset=0  TranslationThetaOffsetUnits=deg  RotationMethod=StandardAxis  RotationAngleUnits=deg  RotationStandardAxis=+Y  RotationAngle=90  RotationArbitraryAxis=[0 0 1]  FollAlignAxisA=+X  BaseAlignAxisA=+Y  FollAlignAxisB=+Y  BaseAlignAxisB=+Z  BlockFunction=simmechanics.library.frames_transforms.rigid_transform
  Rigid Transform1 : sm_lib/Frames and Transforms/Rigid Transform  TranslationMethod=None  TranslationLengthUnit=m  TranslationStandardAxis=+Z  TranslationStandardOffset=0  TranslationCartesianOffset=[0 0 0]  TranslationROffset=0  TranslationROffsetUnits=m  TranslationZOffset=0  TranslationZOffsetUnits=m  TranslationThetaOffset=0  TranslationThetaOffsetUnits=deg  RotationMethod=StandardAxis  RotationAngleUnits=deg  RotationStandardAxis=+Y  RotationAngle=90  RotationArbitraryAxis=[0 0 1]  FollAlignAxisA=+X  BaseAlignAxisA=+Y  FollAlignAxisB=+Y  BaseAlignAxisB=+Z  BlockFunction=simmechanics.library.frames_transforms.rigid_transform
  Selector1 : Selector  InputPortWidth=3  Indices=[3 2 1]
  Selector2 : Selector  InputPortWidth=3  Indices=[3 2 1]
  Selector3 : Selector  InputPortWidth=3  Indices=[3]
  Selector4 : Selector  InputPortWidth=3  Indices=[3]
  Simulink-PS Converter : nesl_utility/Simulink-PS Converter  PhysicalDomain=network_engine_domain  SubClassName=ps_input  LeftPortType=input  RightPortType=output  PseudoPeriodic=off  Frequencies=[]  NoiseDistribution=none  NoiseParameters=[]  Unit=1  AffineConversion=off  InputFiltering=off  SimscapeFilterOrder=1  InputFilterTimeConstant=0.001  UdotUserProvided=1
  Translational PCC (Prismatic Joint) : sm_lib/Joints/Prismatic Joint  SenseConstraintForce=on  SenseConstraintForceX=off  SenseConstraintForceY=off  SenseConstraintForceZ=off  SenseConstraintTorque=on  SenseConstraintTorqueX=off  SenseConstraintTorqueY=off  SenseConstraintTorqueZ=off  SenseTotalForce=off  SenseTotalForceX=off  SenseTotalForceY=off  SenseTotalForceZ=off  SenseTotalTorque=off  SenseTotalTorqueX=off  SenseTotalTorqueY=off  SenseTotalTorqueZ=off  CompositeWrenchDir=BaseOnFollower  CompositeWrenchFrame=BaseFrame  EquilibriumPosition=0  EquilibriumPositionUnits=m  SpringStiffness=0  SpringStiffnessUnits=N/m  DampingCoefficient=0  DampingCoefficientUnits=N/(m/s)  TorqueActuationMode=InputTorque  MotionActuationMode=ComputedMotion  SensePosition=on  SenseVelocity=on  SenseAcceleration=off  SenseTorqueForce=off  PositionTargetValue=0  PositionTargetValueUnits=m  PositionTargetSpecify=off  PositionTargetPriority=High  VelocityTargetValue=0  VelocityTargetValueUnits=m/s  VelocityTargetSpecify=off  VelocityTargetPriority=High  BlockFunction=simmechanics.library.joints.prismatic_joint
  output : ToWorkspace  VariableName=PTO1_out  SaveFormat=Structure With Time  SampleTime=-1
  B : PMIOPort  Port=1  Side=Left
  F : PMIOPort  Port=2  Side=Right
  jointState : Outport
  wires:
  PSS5/1 -> Mux2/2
  PSS/1 -> Mux2/1
  Mux2/1 -> jointState/1
  actuatingForce/1 -> Simulink-PS Converter/1
  Mux/1 -> Mux3/3  "Constraint Forces"
  Selector1/1 -> Assignment/1, Selector4/1
  Selector4/1 -> Gain/1
  Gain/1 -> Assignment/2
  PSS3/1 -> Selector1/1
  Assignment/1 -> Mux/2
  Selector2/1 -> Assignment1/1, Selector3/1
  Selector3/1 -> Gain1/1
  Gain1/1 -> Assignment1/2
  PSS2/1 -> Selector2/1
  Assignment1/1 -> Mux/1
  Constant/1 -> Mux3/1
  Constant1/1 -> Mux3/2
  Mux3/1 -> output/1
  connections:
  Rigid Transform/LConn1 -- B/RConn1
  Rigid Transform/RConn1 -- Translational PCC (Prismatic Joint)/LConn1
  Translational PCC (Prismatic Joint)/RConn1 -- Rigid Transform1/RConn1
  Rigid Transform1/LConn1 -- F/RConn1
  Translational PCC (Prismatic Joint)/RConn2 -- PSS/LConn1
  Translational PCC (Prismatic Joint)/RConn3 -- PSS5/LConn1
  Simulink-PS Converter/RConn1 -- Translational PCC (Prismatic Joint)/LConn2
  Translational PCC (Prismatic Joint)/RConn5 -- PSS3/LConn1
  Translational PCC (Prismatic Joint)/RConn4 -- PSS2/LConn1
